simulink model "MATE_IEEE123Node"  (R2024b)
settings: Solver=FixedStepDiscrete  StartTime=0.0  StopTime=1  FixedStep=Ts  RelTol=1e-3
PostLoadFcn:
  | Ts=50e-6;init_IEEE123Node;
InitFcn:
  | Ts=50e-6;init_IEEE123Node;
values from neighbouring files (symbols this model uses):
  ft2km = 0.0003048    [init_IEEE123Node.m]
  loadcoeff = 1    [init_IEEE123Node.m]
  VsubL = 4.16 * 1000    (= 4160)    [init_IEEE123Node.m]
undefined symbols (not defined in the file or in its folder): MATE, MATERT, Pa1, Pa13, Pa14, Pa17, Pa18, Pa22, Pa24, Pa25, Pa29, Pa31, Pa32, Pa33, Pa34, Pa35, Pa37, Pa38, Pa39, Pa44, Pa46, Pa48, Pa50, Pa51, Pa52, Pa53, Pa57, Pa59, Pa6, Pa61, Pa67, Pa7, Pa70, Pa73, Pa8, Pa81, Pa82, Pa83, Pa84, Pa85, Pa9, Pb10, Pb15, Pb2, Pb30, Pb33, Pb34, Pb35, Pb41, Pb42, Pb43, Pb47, Pb48, Pb57, Pb58, Pb60, Pb65, Pb66, Pb68, Pb71 ... (+121)
libraries: simetranss x259, ee_lib x93, fl_lib x67, nesl_utility x67, simetran x2
(part 1 of 4)
settings Model: ARTEMISmethode_block_infos=$$__separator__$$  Creator=Kyle
settings SolverCC: AlgebraicLoopSolver=TrustRegion
settings DataIOCC: LimitDataPoints=on  SaveFormat=Array  SaveOutput=off  SignalLogging=off  DSMLogging=off  SaveTime=off  ReturnWorkspaceOutputs=off
settings OptimizationCC: OptimizeBlockIOStorage=off  BufferReuse=off  GlobalBufferReuse=off  ExpressionFolding=off  LocalBlockOutputs=off  LifeSpan=inf
settings DebuggingCC: ReadBeforeWriteMsg=DisableAll  WriteAfterWriteMsg=DisableAll  WriteAfterReadMsg=DisableAll  SolverPrmCheckMsg=warning  UnconnectedInputMsg=warning  UnconnectedOutputMsg=warning  UnconnectedLineMsg=warning  AllowSymbolicDim=off  SFUnexpectedBacktrackingDiag=warning  SFNoUnconditionalDefaultTransitionDiag=warning  SFExecutionAtInitializationDiag=none  ArithmeticOperatorsInVariantConditions=warning
settings HardwareCC: ProdBitPerPointer=32  ProdBitPerSizeT=32  ProdBitPerPtrDiffT=32  ProdLargestAtomicFloat=None  ProdIntDivRoundTo=Undefined  ProdEndianess=Unspecified  ProdWordSize=32  ProdHWDeviceType=32-bit Generic
settings ModelReferenceCC: EnableRefExpFcnMdlSchedulingChecks=on  PropagateSignalLabelsOutOfModel=off
settings SFSimCC: SimUseLocalCustomCode=off  CustomCodeUndefinedFunction=UseInterfaceOnly
settings RTWCC: RTWUseLocalCustomCode=off  GPUComputeCapability=3.5
settings CodeAppCC: StateflowObjectComments=on
settings GRTTargetCC: TargetLangStandard=C89/C90 (ANSI)  CombineOutputUpdateFcns=off  GRTInterface=on
settings ConfigComp: CovMetricSettings=dw  CovSaveCumulativeToWorkspaceVar=on  CovSaveSingleToWorkspaceVar=on  CovExternalEMLEnable=off
settings SimscapeCC: SimscapeNormalizeSystem=off

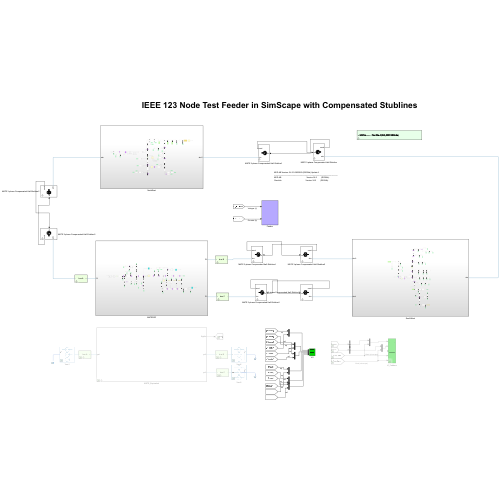
[thumbnail: Simulink's stored preview of the top-level diagram]
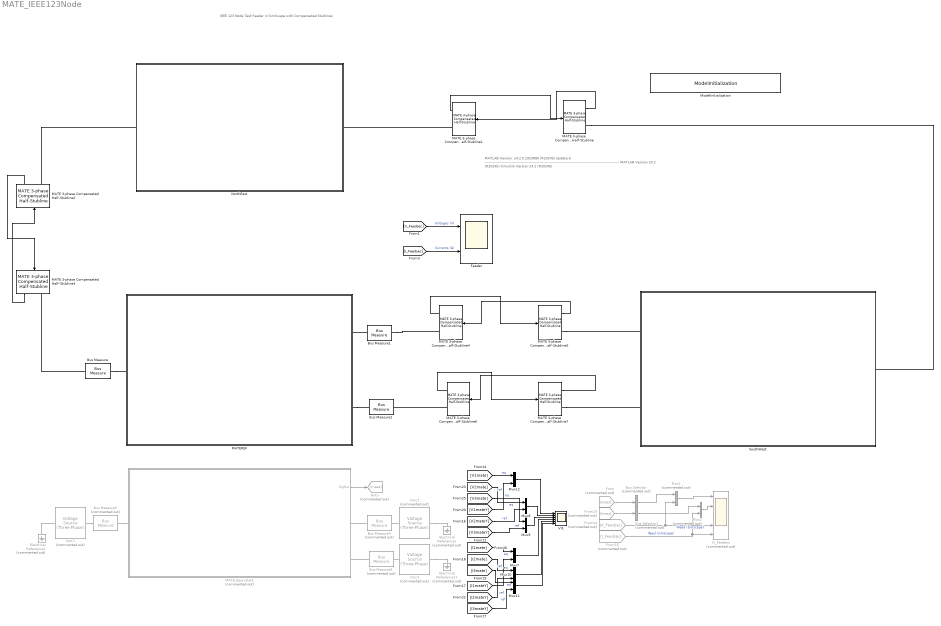
== system MATE_IEEE123Node ==
  note: MATLAB Version: 24.2.0.2923080 (R2024b) Update 6  -----------------------------------------------------------------------------------------------------
      | MATLAB                                                Version 24.2        (R2024b)
      |  Simulink                                              Version 24.2        (R2024b)
  note: IEEE 123 Node Test Feeder in SimScape with Compensated Stublines
  Bus Selector : BusSelector  Commented=on  OutputSignals=Voltage:_5_CV_xfo,Voltage:_6_CV_xfo,Voltage:_7_CV_xfo  OutputAsBus=on
  Bus Selector1 : BusSelector  Commented=on  OutputSignals=current:_11_CV_xfo,current:_12_CV_xfo,current:_13_CV_xfo  OutputAsBus=on
  Bus Measure : simetranss/Measure/Bus Measure  VoltageMeasurement=phase-to-ground  SetLabelV=on  LabelV=V1mateY  Vpu=off  VpuLL=off  CurrentMeasurement=yes  SetLabelI=on  LabelI=I1mateY  Ipu=off  Pbase=100e6  Vbase=500e3  bnumber=A  dis=off
  Bus Measure1 : simetranss/Measure/Bus Measure  VoltageMeasurement=phase-to-ground  SetLabelV=on  LabelV=V2mateY  Vpu=off  VpuLL=off  CurrentMeasurement=yes  SetLabelI=on  LabelI=I2mateY  Ipu=off  Pbase=100e6  Vbase=500e3  bnumber=B  dis=off
  Bus Measure2 : simetranss/Measure/Bus Measure  VoltageMeasurement=phase-to-ground  SetLabelV=on  LabelV=V3mateY  Vpu=off  VpuLL=off  CurrentMeasurement=yes  SetLabelI=on  LabelI=I3mateY  Ipu=off  Pbase=100e6  Vbase=500e3  bnumber=C  dis=off
  Bus Measure3 : simetranss/Measure/Bus Measure  Commented=on  VoltageMeasurement=phase-to-ground  SetLabelV=on  LabelV=V1mate  Vpu=off  VpuLL=off  CurrentMeasurement=yes  SetLabelI=on  LabelI=I1mate  Ipu=off  Pbase=100e6  Vbase=500e3  bnumber=A  dis=off
  Bus Measure4 : simetranss/Measure/Bus Measure  Commented=on  VoltageMeasurement=phase-to-ground  SetLabelV=on  LabelV=V2mate  Vpu=off  VpuLL=off  CurrentMeasurement=yes  SetLabelI=on  LabelI=I2mate  Ipu=off  Pbase=100e6  Vbase=500e3  bnumber=B  dis=off
  Bus Measure5 : simetranss/Measure/Bus Measure  Commented=on  VoltageMeasurement=phase-to-ground  SetLabelV=on  LabelV=V3mate  Vpu=off  VpuLL=off  CurrentMeasurement=yes  SetLabelI=on  LabelI=I3mate  Ipu=off  Pbase=100e6  Vbase=500e3  bnumber=C  dis=off
  Electrical Reference1 : fl_lib/Electrical/Electrical Elements/Electrical Reference  Commented=on
  Electrical Reference11 : fl_lib/Electrical/Electrical Elements/Electrical Reference  Commented=on
  Electrical Reference2 : fl_lib/Electrical/Electrical Elements/Electrical Reference  Commented=on
  Feeder : Scope  NumInputPorts=2
  From : From  Commented=on  GotoTag=meas
  From13 : From  Commented=on  GotoTag=meas
  From14 : From  Commented=on  GotoTag=V_Feedsec  TagVisibility=global
  From15 : From  Commented=on  GotoTag=I_Feedsec  TagVisibility=global
  Goto : Goto  Commented=on  GotoTag=meas
  MATE 3-phase Compensated Half-Stubline : simetranss/Network decoupling/MATE 3-phase Compensated Half-Stubline  stype=3-phase coupled line (1 mode)  FF=60  RR=[ 0.4615 0.1535 0.1580; 0.1535 0.4576 0.1560; 0.1580 0.1560 0.4666]*0.621371  LL=[1.0651 0.3849 0.4236; 0.3849 1.0780 0.5017; 0.4236 0.5017 1.0482]/(2*pi*60)*0.621371  CC=[ 5.3971 -0.6982 -1.1645; -0.6982 5.6765 -1.8319; -1.1645 -1.8319 5.9809]*1e-6/(2*pi*60)*0.621371  len=1000*ft2km  Ts=Ts  comp=on  stdel=off
  MATE 3-phase Compensated Half-Stubline1 : simetranss/Network decoupling/MATE 3-phase Compensated Half-Stubline  stype=3-phase coupled line (1 mode)  FF=60  RR=[ 0.4615 0.1535 0.1580; 0.1535 0.4576 0.1560; 0.1580 0.1560 0.4666]*0.621371  LL=[1.0651 0.3849 0.4236; 0.3849 1.0780 0.5017; 0.4236 0.5017 1.0482]/(2*pi*60)*0.621371  CC=[ 5.3971 -0.6982 -1.1645; -0.6982 5.6765 -1.8319; -1.1645 -1.8319 5.9809]*1e-6/(2*pi*60)*0.621371  len=1000*ft2km  Ts=Ts  comp=off  stdel=off
  MATE 3-phase Compensated Half-Stubline2 : simetranss/Network decoupling/MATE 3-phase Compensated Half-Stubline  stype=3-phase coupled line (1 mode)  FF=60  RR=[ 0.4666 0.1580 0.1560; 0.1580 0.4615 0.1535; 0.1560 0.1535 0.4576]*0.621371  LL=[ 1.0482 0.4236 0.5017; 0.4236 1.0651 0.3849; 0.5017 0.3849 1.0780]/(2*pi*60)*0.621371  CC=[ 5.9809 -1.1645 -1.8319; -1.1645 5.3971 -0.6982; -1.8319 -0.6982 5.6765]*1e-6/(2*pi*60)*0.621371  len=825*ft2km  Ts=Ts  comp=on  stdel=off
  MATE 3-phase Compensated Half-Stubline3 : simetranss/Network decoupling/MATE 3-phase Compensated Half-Stubline  stype=3-phase coupled line (1 mode)  FF=60  RR=[ 0.4666 0.1580 0.1560; 0.1580 0.4615 0.1535; 0.1560 0.1535 0.4576]*0.621371  LL=[ 1.0482 0.4236 0.5017; 0.4236 1.0651 0.3849; 0.5017 0.3849 1.0780]/(2*pi*60)*0.621371  CC=[ 5.9809 -1.1645 -1.8319; -1.1645 5.3971 -0.6982; -1.8319 -0.6982 5.6765]*1e-6/(2*pi*60)*0.621371  len=825*ft2km  Ts=Ts  comp=off  stdel=off
  MATE 3-phase Compensated Half-Stubline4 : simetranss/Network decoupling/MATE 3-phase Compensated Half-Stubline  stype=3-phase coupled line (1 mode)  FF=60  RR=[ 0.4615 0.1535 0.1580; 0.1535 0.4576 0.1560; 0.1580 0.1560 0.4666]*0.621371  LL=[1.0651 0.3849 0.4236; 0.3849 1.0780 0.5017; 0.4236 0.5017 1.0482]/(2*pi*60)*0.621371  CC=[ 5.3971 -0.6982 -1.1645; -0.6982 5.6765 -1.8319; -1.1645 -1.8319 5.9809]*1e-6/(2*pi*60)*0.621371  len=750*ft2km  Ts=Ts  comp=off  stdel=off
  MATE 3-phase Compensated Half-Stubline5 : simetranss/Network decoupling/MATE 3-phase Compensated Half-Stubline  stype=3-phase coupled line (1 mode)  FF=60  RR=[ 0.4615 0.1535 0.1580; 0.1535 0.4576 0.1560; 0.1580 0.1560 0.4666]*0.621371  LL=[1.0651 0.3849 0.4236; 0.3849 1.0780 0.5017; 0.4236 0.5017 1.0482]/(2*pi*60)*0.621371  CC=[ 5.3971 -0.6982 -1.1645; -0.6982 5.6765 -1.8319; -1.1645 -1.8319 5.9809]*1e-6/(2*pi*60)*0.621371  len=750*ft2km  Ts=Ts  comp=on  stdel=off
  MATE 3-phase Compensated Half-Stubline6 : simetranss/Network decoupling/MATE 3-phase Compensated Half-Stubline  stype=3-phase coupled line (1 mode)  FF=60  RR=[ 0.4615 0.1535 0.1580; 0.1535 0.4576 0.1560; 0.1580 0.1560 0.4666]*0.621371  LL=[1.0651 0.3849 0.4236; 0.3849 1.0780 0.5017; 0.4236 0.5017 1.0482]/(2*pi*60)*0.621371  CC=[ 5.3971 -0.6982 -1.1645; -0.6982 5.6765 -1.8319; -1.1645 -1.8319 5.9809]*1e-6/(2*pi*60)*0.621371  len=700*ft2km  Ts=Ts  comp=on  stdel=off
  MATE 3-phase Compensated Half-Stubline7 : simetranss/Network decoupling/MATE 3-phase Compensated Half-Stubline  stype=3-phase coupled line (1 mode)  FF=60  RR=[ 0.4615 0.1535 0.1580; 0.1535 0.4576 0.1560; 0.1580 0.1560 0.4666]*0.621371  LL=[1.0651 0.3849 0.4236; 0.3849 1.0780 0.5017; 0.4236 0.5017 1.0482]/(2*pi*60)*0.621371  CC=[ 5.3971 -0.6982 -1.1645; -0.6982 5.6765 -1.8319; -1.1645 -1.8319 5.9809]*1e-6/(2*pi*60)*0.621371  len=700*ft2km  Ts=Ts  comp=off  stdel=off
  MATEREF : Subsystem
  MATE_Equivalent : Subsystem  Commented=on  mask(MATE object){MATE=MATE, MATERT=MATERT}
      mask prompts: MATE "General MATE data structure name"; MATERT "MATE S-function parameter"
      mask help:
      | MATE Object (Multu-Area Thevenin Equivalent) is a generalized EMT-type branch.
      | They can be used to build equivalent circuit with less solver apparent nodes.
      mask DialogControl Control2 Prompt: Generate MATE equations
      mask DialogControl Control2 Callback:
      | [MATE, MATERT]= MakeMate('Simscape_IEEE123_oneThird/MATEREF', 1);
      | assignin("base","MATE",MATE);
      | assignin("base","MATERT",MATERT);
  ModelInitialization : simetranss/Usefulls/ModelInitialization  InitFcnX=Ts=50e-6;init_IEEE123Node;  prel=off  posl=on  inif=on  strf=off
  Mux1 : Mux  Commented=on  Inputs=2
  Mux{7..12} (6 alike) : Mux  Inputs=2
  Mux2 : Mux  Commented=on  Inputs=2
  NorthEast : Subsystem
  SouthWest : Subsystem
  VI1 : Scope  NumInputPorts=6
  VI_Fedders : Scope  Commented=on  NumInputPorts=5
  Vsrc1 : ee_lib/Sources/Voltage Source (Three-Phase)  Commented=on  vline_rms=4160 V  shift=0 deg  freq=60 Hz  impedance_option=4  SShortCircuit=1e6 A*V  XR=15  R=0.1 Ohm  L=1e-3 H  harmonic_option=0  harmonic_orders=[5, 7, 11, 13]  harmonic_ratios=[.1, .1, .1, .1]  G_parasitic=0 1/Ohm  I_specify=off  I_priority=None  I=[0, 0, 0] A  I_nominal_specify=off  I_nominal_value=1  I_nominal_unit=A
  Vsrc2 : ee_lib/Sources/Voltage Source (Three-Phase)  Commented=on  vline_rms=4160 V  shift=15 deg  freq=60 Hz  impedance_option=4  SShortCircuit=1e6 A*V  XR=15  R=0.1 Ohm  L=1e-3 H  harmonic_option=0  harmonic_orders=[5, 7, 11, 13]  harmonic_ratios=[.1, .1, .1, .1]  G_parasitic=0 1/Ohm  I_specify=off  I_priority=None  I=[0, 0, 0] A  I_nominal_specify=off  I_nominal_value=1  I_nominal_unit=A
  Vsrc3 : ee_lib/Sources/Voltage Source (Three-Phase)  Commented=on  vline_rms=4160 V  shift=30 deg  freq=60 Hz  impedance_option=4  SShortCircuit=1e6 A*V  XR=15  R=0.1 Ohm  L=1e-3 H  harmonic_option=0  harmonic_orders=[5, 7, 11, 13]  harmonic_ratios=[.1, .1, .1, .1]  G_parasitic=0 1/Ohm  I_specify=off  I_priority=None  I=[0, 0, 0] A  I_nominal_specify=off  I_nominal_value=1  I_nominal_unit=A
  wires:
  [I2mateY] -> Mux10/2  "ref"
  [I1mate] -> Mux7/1  "eq"
  From13/1 -> Bus Selector1/1
  From/1 -> Bus Selector/1
  Mux9/1 -> VI1/3
  [V2mate] -> Mux8/1  "eq"
  [V3mateY] -> Mux9/2  "ref"
  Bus Selector1/1 -> Mux2/1
  Mux11/1 -> VI1/6
  Mux12/1 -> VI1/1
  Mux10/1 -> VI1/5
  [I2mate] -> Mux10/1  "eq"
  [V3mate] -> Mux9/1  "eq"
  Mux7/1 -> VI1/4
  [V1mate] -> Mux12/1  "eq"
  [I3mateY] -> Mux11/2  "ref"
  [I3mate] -> Mux11/1  "eq"
  [I1mateY] -> Mux7/2  "ref"
  From14/1 -> Mux1/2, VI_Fedders/4  "Vfeed (simscape)"
  Mux1/1 -> VI_Fedders/1
  Mux8/1 -> VI1/2
  Bus Selector/1 -> Mux1/1
  Mux2/1 -> VI_Fedders/2
  [V1mateY] -> Mux12/2  "ref"
  From15/1 -> Mux2/2, VI_Fedders/5  "Ifeed (simscape)"
  MATE_Equivalent/1(SigOut) -> Goto/1
  [V2mateY] -> Mux8/2  "ref"
  MATE 3-phase Compensated Half-Stubline/1 -> MATE 3-phase Compensated Half-Stubline1/1
  MATE 3-phase Compensated Half-Stubline1/1 -> MATE 3-phase Compensated Half-Stubline/1
  MATE 3-phase Compensated Half-Stubline2/1 -> MATE 3-phase Compensated Half-Stubline3/1
  MATE 3-phase Compensated Half-Stubline3/1 -> MATE 3-phase Compensated Half-Stubline2/1
  MATE 3-phase Compensated Half-Stubline4/1 -> MATE 3-phase Compensated Half-Stubline5/1
  MATE 3-phase Compensated Half-Stubline5/1 -> MATE 3-phase Compensated Half-Stubline4/1
  MATE 3-phase Compensated Half-Stubline6/1 -> MATE 3-phase Compensated Half-Stubline7/1
  MATE 3-phase Compensated Half-Stubline7/1 -> MATE 3-phase Compensated Half-Stubline6/1
  [V_Feedsec] -> Feeder/1  "Voltages (V)"
  [I_Feedsec] -> Feeder/2  "Currents (A)"
  connections:
  MATE 3-phase Compensated Half-Stubline6/RConn1 -- Bus Measure2/RConn1
  Bus Measure1/RConn1 -- MATE 3-phase Compensated Half-Stubline4/RConn1
  Bus Measure/RConn1 -- MATE 3-phase Compensated Half-Stubline3/RConn1
  Bus Measure/LConn1 -- MATEREF/LConn1
  MATEREF/RConn2 -- Bus Measure2/LConn1
  Vsrc3/LConn1 -- Electrical Reference11/LConn1
  Vsrc1/LConn1 -- Electrical Reference2/LConn1
  Vsrc3/RConn1 -- Bus Measure5/RConn1
  Vsrc2/LConn1 -- Electrical Reference1/LConn1
  Bus Measure1/LConn1 -- MATEREF/RConn1
  MATE 3-phase Compensated Half-Stubline1/RConn1 -- NorthEast/RConn1
  MATE 3-phase Compensated Half-Stubline/RConn1 -- SouthWest/RConn1
  MATE 3-phase Compensated Half-Stubline5/RConn1 -- SouthWest/LConn1
  MATE 3-phase Compensated Half-Stubline7/RConn1 -- SouthWest/LConn2
  Bus Measure3/LConn1 -- MATE_Equivalent/LConn1
  Bus Measure4/LConn1 -- MATE_Equivalent/RConn1
  NorthEast/LConn1 -- MATE 3-phase Compensated Half-Stubline2/RConn1
  Vsrc1/RConn1 -- Bus Measure3/RConn1
  Vsrc2/RConn1 -- Bus Measure4/RConn1
  Bus Measure5/LConn1 -- MATE_Equivalent/RConn2

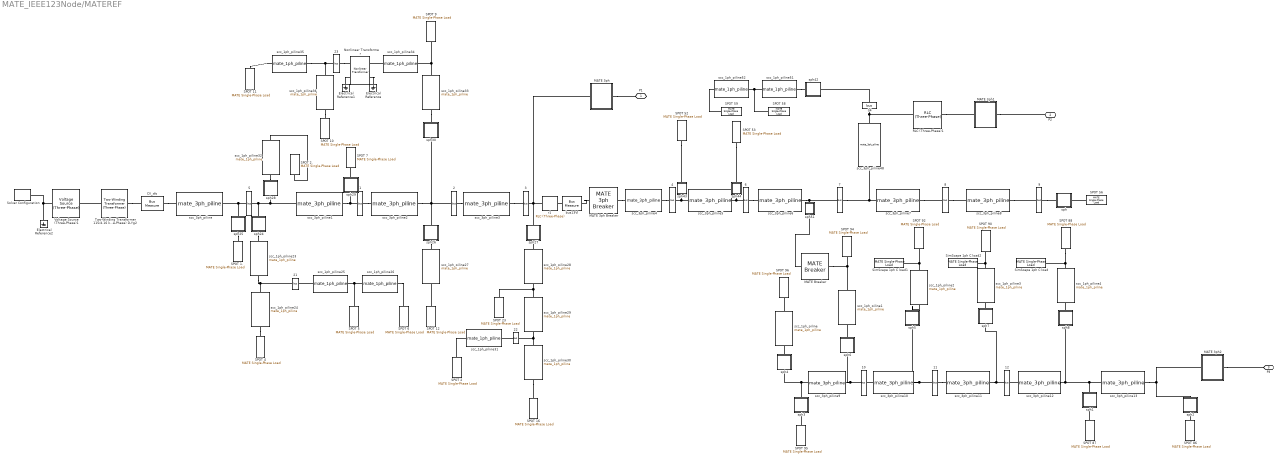
== system MATE_IEEE123Node/MATEREF ==
  1 : simetranss/Measure/bus  bn=7
      settings: AttributesFormatString=Bus %<bn>
  10 : simetranss/Measure/bus  bn=93
      settings: AttributesFormatString=Bus %<bn>
  11 : simetranss/Measure/bus  bn=91
      settings: AttributesFormatString=Bus %<bn>
  12 : simetranss/Measure/bus  bn=89
      settings: AttributesFormatString=Bus %<bn>
  2 : simetranss/Measure/bus  bn=8
      settings: AttributesFormatString=Bus %<bn>
  21 : simetranss/Measure/bus  bn=3
      settings: AttributesFormatString=Bus %<bn>
  22 : simetranss/Measure/bus  bn=15
      settings: AttributesFormatString=Bus %<bn>
  23 : simetranss/Measure/bus  bn=14
      settings: AttributesFormatString=Bus %<bn>
  3 : simetranss/Measure/bus  bn=13
      settings: AttributesFormatString=Bus %<bn>
  34 : simetranss/Measure/bus  bn=57
      settings: AttributesFormatString=Bus %<bn>
  4 : simetranss/Measure/bus  bn=52
      settings: AttributesFormatString=Bus %<bn>
  5 : simetranss/Measure/bus  bn=1
      settings: AttributesFormatString=Bus %<bn>
  6 : simetranss/Measure/bus  bn=53
      settings: AttributesFormatString=Bus %<bn>
  7 : simetranss/Measure/bus  bn=54
      settings: AttributesFormatString=Bus %<bn>
  8 : simetranss/Measure/bus  bn=55
      settings: AttributesFormatString=Bus %<bn>
  9 : simetranss/Measure/bus  bn=56
      settings: AttributesFormatString=Bus %<bn>
  CV_xfo : simetranss/Measure/Bus Measure  VoltageMeasurement=phase-to-ground  SetLabelV=on  LabelV=V_Feedsec  Vpu=off  VpuLL=off  CurrentMeasurement=yes  SetLabelI=on  LabelI=I_Feedsec  Ipu=off  Pbase=100e6  Vbase=500e3  bnumber=0  dis=off
  Electrical Reference : fl_lib/Electrical/Electrical Elements/Electrical Reference
  Electrical Reference1 : fl_lib/Electrical/Electrical Elements/Electrical Reference
  Electrical Reference2 : fl_lib/Electrical/Electrical Elements/Electrical Reference
  MATE 3ph : Subsystem  mask(MATE Node (3-phase)){bn=1, it=auto, Rse=1e-4, Rsh=1e9}
      mask prompts: bn "MATE node number"; it "Interface type"; Rse "Series resistance (Ohms)"; Rsh "Shunt resistance (Ohms)"
      mask help:
      | MATE interface for Single-Line Diagram SimScape model.
      |
      | This block is used to interface a MATE reduced set of block to a main circuit.
      | 'MATE' port must be connected toward the MATE reduced network.
      | 'Main' port must be connected toward the main (unreduced) network)
      settings: AttributesFormatString=# %<bn>
      mask TypeOptions it: auto | Thevenin | Norton
      mask Display: disp(['3ph' 10 10 10])
  MATE 3ph Breaker : simetranss/Switches/MATE 3ph Breaker  InitialState=closed  SwitchA=off  SwitchB=off  SwitchC=off  SwitchTimes="[1/60  5/60]"  External=off  BreakerResistance=0.01  Roff=0  SnubberResistance=1e6  SnubberCapacitance=inf
  MATE 3ph1 : Subsystem  mask(MATE Node (3-phase)){bn=2, it=auto, Rse=1e-4, Rsh=1e9}
      mask prompts: bn "MATE node number"; it "Interface type"; Rse "Series resistance (Ohms)"; Rsh "Shunt resistance (Ohms)"
      mask help:
      | MATE interface for Single-Line Diagram SimScape model.
      |
      | This block is used to interface a MATE reduced set of block to a main circuit.
      | 'MATE' port must be connected toward the MATE reduced network.
      | 'Main' port must be connected toward the main (unreduced) network)
      settings: AttributesFormatString=# %<bn>
      mask TypeOptions it: auto | Thevenin | Norton
      mask Display: disp(['3ph' 10 10 10])
  MATE 3ph2 : Subsystem  mask(MATE Node (3-phase)){bn=3, it=auto, Rse=1e-4, Rsh=1e9}
      mask prompts: bn "MATE node number"; it "Interface type"; Rse "Series resistance (Ohms)"; Rsh "Shunt resistance (Ohms)"
      mask help:
      | MATE interface for Single-Line Diagram SimScape model.
      |
      | This block is used to interface a MATE reduced set of block to a main circuit.
      | 'MATE' port must be connected toward the MATE reduced network.
      | 'Main' port must be connected toward the main (unreduced) network)
      settings: AttributesFormatString=# %<bn>
      mask TypeOptions it: auto | Thevenin | Norton
      mask Display: disp(['3ph' 10 10 10])
  MATE Breaker : simetranss/Switches/MATE Breaker  InitialState=open  SwitchA=on  SwitchB=on  SwitchC=off  SwitchTimes="[1/60  5/60]"  External=off  BreakerResistance=0.01  Roff=1e6  SnubberResistance=1e6  SnubberCapacitance=inf
  Nonlinear Transformer : ee_lib/Passive/Transformers/Nonlinear Transformer  Nw=1  Nw2=1  winding_param_option=2  Req=0.01 Ohm  Leq=0.0001 H  R_1=0.001 Ohm  L_1=0.001 H  R_2=0.001 Ohm  L_2=0.001 H  averaging_period=0 s  R_m=50000 Ohm  parameterization_option=1  H_data=[0, 200, 400, 600, 800, 1000] A/m  B_data=[0, .81, 1.25, 1.42, 1.48, 1.49] T  length_effective=0.2 m  area_effective=2e-4 m^2  L=4e-2 H  L_sat=1e-2 H  current_data=[0, .4, .8, 1.2, 1.6, 2] A  magnetic_flux_data=[0, .161, .25, .284, .295, .299] .* 1e-3 Wb  magnetic_flux_sat=1.6e-04 Wb  dBdH0=0.005 T*m/A  B1=1.49 T  H1=1000 A/m  c=0.1  K=200 A/m  alpha=1e-4  interpolation_option=1  Leq_i0=0 A  L1_i0=0 A  L2_i0=0 A  x0_option=1  i_L0=0 A  phi0=0 Wb  B0=0 T  H0=0 A/m  Leq_g=1e-9 1/Ohm  L1_g=1e-9 1/Ohm  L2_g=1e-9 1/Ohm
      settings: InternalSimscapePortConfiguration="{\"Bottom\":[],\"Left\":[{\"id\":\"p1\",\"label\":\"1+\",\"type\":\"foundation.electrical.electrical\"},{\"id\":\"n1\",\"label\":\"1-\",\"type\":\"foundation.electrical.electrical\"}],\"Right\":[{\"id\":\"p2\",\"label\":\"2+\",\"type\":\"foundation.electrical.electrical\"},{\"id\":\"n2\",\"label\":\"2-\",\"type\":\"foundation.electrical.electrical\"}],\"Top\":[]}"
  RLC (Three-Phase)1 : ee_lib/Passive/RLC Assemblies/RLC (Three-Phase)  port_option=ee.enum.threePhasePort.composite  component_structure=ee.enum.rlc.structure.SeriesRL  R=1e-2 Ohm  L=1e-6 H  C=1e-6 F  R_parasitic=0 Ohm  G_parasitic=0 1/Ohm  IL_specify=off  IL_priority=High  IL=[0, 0, 0] A  IL_nominal_specify=off  IL_nominal_value=1  IL_nominal_unit=A  VC_specify=off  VC_priority=High  VC=[0, 0, 0] V  VC_nominal_specify=off  VC_nominal_value=1  VC_nominal_unit=V
      settings: InternalSimscapePortConfiguration="{\"Bottom\":[],\"Left\":[{\"id\":\"N1\",\"label\":\"~1\",\"type\":\"foundation.electrical.three_phase\"}],\"Right\":[{\"id\":\"N2\",\"label\":\"~2\",\"type\":\"foundation.electrical.three_phase\"}],\"Top\":[]}"
  SPOT 1. : simetranss/Passive/MATE Single-Phase Load  Vabc=VsubL/sqrt(3)  Fn=60  typ=Series RL  Pabc=Pa1*loadcoeff  QLabc=Qa1*loadcoeff  QCabc="[190  ]*1e3"
  SPOT 10 : simetranss/Passive/MATE Single-Phase Load  Vabc=VsubL/sqrt(3)  Fn=60  typ=Series RL  Pabc=Pa8*loadcoeff  QLabc=Qa8*loadcoeff  QCabc="[190  ]*1e3"
  SPOT 11 : simetranss/Passive/MATE Single-Phase Load  Vabc=VsubL/sqrt(3)  Fn=60  typ=Series RL  Pabc=Pa9*loadcoeff  QLabc=Qa9*loadcoeff  QCabc="[190  ]*1e3"
  SPOT 12 : simetranss/Passive/MATE Single-Phase Load  Vabc=VsubL/sqrt(3)  Fn=60  typ=Series RL  Pabc=Pb10*loadcoeff  QLabc=Qb10*loadcoeff  QCabc="[190  ]*1e3"
  SPOT 16 : simetranss/Passive/MATE Single-Phase Load  Vabc=VsubL/sqrt(3)  Fn=60  typ=Series RL  Pabc=Pc11*loadcoeff  QLabc=Qc11*loadcoeff  QCabc="[190  ]*1e3"
  SPOT 2 : simetranss/Passive/MATE Single-Phase Load  Vabc=VsubL/sqrt(3)  Fn=60  typ=Series RL  Pabc=Pc12*loadcoeff  QLabc=Qc12*loadcoeff  QCabc="[190  ]*1e3"
  SPOT 2. : simetranss/Passive/MATE Single-Phase Load  Vabc=VsubL/sqrt(3)  Fn=60  typ=Series RL  Pabc=Pb2*loadcoeff  QLabc=Qb2*loadcoeff  QCabc="[190  ]*1e3"
  SPOT 23 : simetranss/Passive/MATE Single-Phase Load  Vabc=VsubL/sqrt(3)  Fn=60  typ=Series RL  Pabc=Pc11*loadcoeff  QLabc=Qc11*loadcoeff  QCabc="[190  ]*1e3"
  SPOT 4 : simetranss/Passive/MATE Single-Phase Load  Vabc=VsubL/sqrt(3)  Fn=60  typ=Series RL  Pabc=Pc3*loadcoeff  QLabc=Qc3*loadcoeff  QCabc="[190  ]*1e3"
  SPOT 5 : simetranss/Passive/MATE Single-Phase Load  Vabc=VsubL/sqrt(3)  Fn=60  typ=Series RL  Pabc=Pc4*loadcoeff  QLabc=Qc4*loadcoeff  QCabc="[190  ]*1e3"
  SPOT 52 : simetranss/Passive/MATE Single-Phase Load  Vabc=VsubL/sqrt(3)  Fn=60  typ=Series RL  Pabc=Pa38*loadcoeff  QLabc=Qa38*loadcoeff  QCabc="[190  ]*1e3"
  SPOT 53 : simetranss/Passive/MATE Single-Phase Load  Vabc=VsubL/sqrt(3)  Fn=60  typ=Series RL  Pabc=Pa39*loadcoeff  QLabc=Qa39*loadcoeff  QCabc="[190  ]*1e3"
  SPOT 56 : simetranss/Passive/MATE Single-Phase Load  Vabc=VsubL/sqrt(3)  Fn=60  typ=Series RL  Pabc=Pb41*loadcoeff  QLabc=Qb41*loadcoeff  QCabc="[190  ]*1e3"
  SPOT 58 : simetranss/Passive/MATE Single-Phase Load  Vabc=VsubL/sqrt(3)  Fn=60  typ=Series RL  Pabc=Pb42*loadcoeff  QLabc=Qb42*loadcoeff  QCabc="[190  ]*1e3"
  SPOT 59 : simetranss/Passive/MATE Single-Phase Load  Vabc=VsubL/sqrt(3)  Fn=60  typ=Series RL  Pabc=Pb43*loadcoeff  QLabc=Qb43*loadcoeff  QCabc="[190  ]*1e3"
  SPOT 6 : simetranss/Passive/MATE Single-Phase Load  Vabc=VsubL/sqrt(3)  Fn=60  typ=Series RL  Pabc=Pc5*loadcoeff  QLabc=Qc5*loadcoeff  QCabc="[190  ]*1e3"
  SPOT 7 : simetranss/Passive/MATE Single-Phase Load  Vabc=VsubL/sqrt(3)  Fn=60  typ=Series RL  Pabc=Pa6*loadcoeff  QLabc=Qa6*loadcoeff  QCabc="[190  ]*1e3"
  SPOT 86 : simetranss/Passive/MATE Single-Phase Load  Vabc=VsubL/sqrt(3)  Fn=60  typ=Series RL  Pabc=Pb65*loadcoeff  QLabc=Qb65*loadcoeff  QCabc="[190  ]*1e3"
  SPOT 87 : simetranss/Passive/MATE Single-Phase Load  Vabc=VsubL/sqrt(3)  Fn=60  typ=Series RL  Pabc=Pb66*loadcoeff  QLabc=Qb66*loadcoeff  QCabc="[190  ]*1e3"
  SPOT 88 : simetranss/Passive/MATE Single-Phase Load  Vabc=VsubL/sqrt(3)  Fn=60  typ=Series RL  Pabc=Pa67*loadcoeff  QLabc=Qa67*loadcoeff  QCabc="[190  ]*1e3"
  SPOT 9 : simetranss/Passive/MATE Single-Phase Load  Vabc=VsubL/sqrt(3)  Fn=60  typ=Series RL  Pabc=Pa7*loadcoeff  QLabc=Qa7*loadcoeff  QCabc="[190  ]*1e3"
  SPOT 90 : simetranss/Passive/MATE Single-Phase Load  Vabc=VsubL/sqrt(3)  Fn=60  typ=Series RL  Pabc=Pb68*loadcoeff  QLabc=Qb68*loadcoeff  QCabc="[190  ]*1e3"
  SPOT 92 : simetranss/Passive/MATE Single-Phase Load  Vabc=VsubL/sqrt(3)  Fn=60  typ=Series RL  Pabc=Pc69*loadcoeff  QLabc=Qc69*loadcoeff  QCabc="[190  ]*1e3"
  SPOT 94 : simetranss/Passive/MATE Single-Phase Load  Vabc=VsubL/sqrt(3)  Fn=60  typ=Series RL  Pabc=Pa70*loadcoeff  QLabc=Qa70*loadcoeff  QCabc="[190  ]*1e3"
  SPOT 95 : simetranss/Passive/MATE Single-Phase Load  Vabc=VsubL/sqrt(3)  Fn=60  typ=Series RL  Pabc=Pb71*loadcoeff  QLabc=Qb71*loadcoeff  QCabc="[190  ]*1e3"
  SPOT 96 : simetranss/Passive/MATE Single-Phase Load  Vabc=VsubL/sqrt(3)  Fn=60  typ=Series RL  Pabc=Pb72*loadcoeff  QLabc=Qb72*loadcoeff  QCabc="[190  ]*1e3"
  SimScape 1ph C load : simetranss/Passive/MATE Single-Phase Load  Vabc=4160/sqrt(3)  Fn=60  typ=Capacitance  Pabc=[160 ]*1e3  QLabc=[ 90]*1e3  QCabc=100e3
  SimScape 1ph C load1 : simetranss/Passive/MATE Single-Phase Load  Vabc=VsubL/sqrt(3)  Fn=60  typ=Capacitance  Pabc=[160 ]*1e3  QLabc=[ 90]*1e3  QCabc=50e3
  SimScape 1ph C load2 : simetranss/Passive/MATE Single-Phase Load  Vabc=VsubL/sqrt(3)  Fn=60  typ=Capacitance  Pabc=[160 ]*1e3  QLabc=[ 90]*1e3  QCabc=50e3
  Solver Configuration : nesl_utility/Solver Configuration  PhysicalDomain=network_engine_domain  SubClassName=solver  LeftPortType=input  RightPortType=generic  Tones=[]  Harmonics=[]  SimulateNoise=off  Profile=off  UseLocalSampling=off  EnableSwitchedLinearOptims=on  FrequencyDomain=off  UseCCode=off  RelTol=0.001  AbsTol=0.001  MinStep=1e-09  ToWorkspace=off  RevertToSquareIcSolve=off  NumHomotopyIterations=100  PhasorMode=off  PhasorModeNumHarmonics=1  ConsistencySolver=NEWTON_XTOL_AFTER_FTOL  IndexReductionMethod=None  DoDC=off  ResidualTolerance=1e-09  ConsistencyTolSource=GLOBAL  ConsistencyAbsTol=0.001  ConsistencyRelTol=0.001  ConsistencyTolFactor=0.1  UseLocalSolver=on  LocalSolverChoice=NE_PARTITIONING_ADVANCER  ResolveIndetEquations=off  FunctionEvalNumThread=1  LocalSolverSampleTime=Ts  DoFixedCost=on  MaxNonlinIter=1  MaxModeIter=2  ComputeImpulses=off  ImpulseIterations=2  LinearAlgebra=auto  LinearAlgebraNumThread=0  EquationFormulation=NE_TIME_EF  DelaysMemoryBudget=1024  AutomaticFiltering=on  FilteringTimeConstant=0.001  PartitionStorageMethod=AS_NEEDED  PartitionMemoryBudget=1024  PartitionMethod=ROBUST  MultibodyUseLocalSolver=off  MultibodyLocalSolverChoice=ODE1  MultibodyLocalSolverSampleTime=0.001
  Two-Winding Transformer 115/4.16 kV (Three-Phase) D-Yg2 : ee_lib/Passive/Transformers/Two-Winding Transformer (Three-Phase)  SRated=6e6 A*V  FRated=60 Hz  Winding1Connection=ee.enum.windingconnection.delta1  VRated1=115e3 V  Winding2Connection=ee.enum.windingconnection.Yg  VRated2=4160 V  CoreType=ee.enum.coretype.fivelimb  pu_Rw1=0.01/2  pu_Rw2=0.01/2  leakage_reactance_option=ee.enum.transformer_leakage.include  pu_Xl1=0.08/2  pu_Xl2=0.08/2  magnetizing_resistance_option=ee.enum.transformer_magnetizingResistance.include  pu_Rm=100  magnetizing_reactance_option=ee.enum.transformer_magnetizingReactance.include  saturation_option=ee.enum.transformer_saturation.exclude  pu_Xm=100  current_data=[0, .002, 1, 2]  magnetic_flux_data=[0, 1.2, 1.5, 1.51]  pu_X0=5000  i1_specify=off  i1_priority=None  i1=[0, 0, 0] A  i1_nominal_specify=off  i1_nominal_value=1  i1_nominal_unit=A  i2_specify=off  i2_priority=None  i2=[0, 0, 0] A  i2_nominal_specify=off  i2_nominal_value=1  i2_nominal_unit=A  phi_specify=off  phi_priority=None  phi=[0, 0, 0]  phi_nominal_specify=off  phi_nominal_value=1  phi_nominal_unit=1  power_dissipated_specify=off  power_dissipated_priority=None  power_dissipated=0 W  power_dissipated_nominal_specify=off  power_dissipated_nominal_value=1  power_dissipated_nominal_unit=W
      settings: InternalSimscapePortConfiguration="{\"Bottom\":[],\"Left\":[{\"id\":\"N1\",\"label\":\"~1\",\"type\":\"foundation.electrical.three_phase\"}],\"Right\":[{\"id\":\"N2\",\"label\":\"~2\",\"type\":\"foundation.electrical.three_phase\"}],\"Top\":[]}"
  Voltage Source (Three-Phase)1 : ee_lib/Sources/Voltage Source (Three-Phase)  vline_rms=115e3 V  shift=90 deg  freq=60 Hz  impedance_option=2  SShortCircuit=1e6 A*V  XR=15  R=0.001 Ohm  L=3.97e-4 H  harmonic_option=0  harmonic_orders=[5, 7, 11, 13]  harmonic_ratios=[.1, .1, .1, .1]  G_parasitic=0 1/Ohm  I_specify=off  I_priority=None  I=[0, 0, 0] A  I_nominal_specify=off  I_nominal_value=1  I_nominal_unit=A
  bus13VI : simetranss/Measure/Bus Measure  VoltageMeasurement=phase-to-ground  SetLabelV=on  LabelV=V13  Vpu=off  VpuLL=off  CurrentMeasurement=yes  SetLabelI=on  LabelI=I13  Ipu=off  Pbase=100e6  Vbase=500e3  bnumber=13  dis=off
  r1 : ee_lib/Passive/RLC Assemblies/RLC (Three-Phase)  port_option=ee.enum.threePhasePort.composite  component_structure=ee.enum.rlc.structure.R  R=1e-3 Ohm  L=1e-3 H  C=1e-6 F  R_parasitic=0 Ohm  G_parasitic=0 1/Ohm  IL_specify=off  IL_priority=High  IL=[0, 0, 0] A  IL_nominal_specify=off  IL_nominal_value=1  IL_nominal_unit=A  VC_specify=off  VC_priority=High  VC=[0, 0, 0] V  VC_nominal_specify=off  VC_nominal_value=1  VC_nominal_unit=V
      settings: InternalSimscapePortConfiguration="{\"Bottom\":[],\"Left\":[{\"id\":\"N1\",\"label\":\"~1\",\"type\":\"foundation.electrical.three_phase\"}],\"Right\":[{\"id\":\"N2\",\"label\":\"~2\",\"type\":\"foundation.electrical.three_phase\"}],\"Top\":[]}"
  scc_1ph_piline : simetranss/Lines/mate_1ph_piline  FF=60  conf=config 10  lenfeet=200  dmi=off  RR1=0.8  LL1=0.002  CC1=7e-9  lenkm=300*ft2km
  scc_1ph_piline1 : simetranss/Lines/mate_1ph_piline  FF=60  conf=config 9  lenfeet=275  dmi=off  RR1=0.8  LL1=0.002  CC1=7e-9  lenkm=300*ft2km
  scc_1ph_piline2 : simetranss/Lines/mate_1ph_piline  FF=60  conf=config 11  lenfeet=300  dmi=off  RR1=0.8  LL1=0.002  CC1=7e-9  lenkm=300*ft2km
  scc_1ph_piline23 : simetranss/Lines/mate_1ph_piline  FF=60  conf=config 11  lenfeet=250  dmi=off  RR1=0.8  LL1=0.002  CC1=7e-9  lenkm=1
  scc_1ph_piline24 : simetranss/Lines/mate_1ph_piline  FF=60  conf=config 11  lenfeet=200  dmi=off  RR1=0.8  LL1=0.002  CC1=7e-9  lenkm=1
  scc_1ph_piline25 : simetranss/Lines/mate_1ph_piline  FF=60  conf=config 11  lenfeet=325  dmi=off  RR1=0.8  LL1=0.002  CC1=7e-9  lenkm=1
  scc_1ph_piline26 : simetranss/Lines/mate_1ph_piline  FF=60  conf=config 11  lenfeet=250  dmi=off  RR1=0.8  LL1=0.002  CC1=7e-9  lenkm=1
  scc_1ph_piline27 : simetranss/Lines/mate_1ph_piline  FF=60  conf=config 10  lenfeet=225  dmi=off  RR1=0.8  LL1=0.002  CC1=7e-9  lenkm=1
  scc_1ph_piline28 : simetranss/Lines/mate_1ph_piline  FF=60  conf=config 11  lenfeet=150  dmi=off  RR1=0.8  LL1=0.002  CC1=7e-9  lenkm=1
  scc_1ph_piline29 : simetranss/Lines/mate_1ph_piline  FF=60  conf=config 11  lenfeet=100  dmi=off  RR1=0.8  LL1=0.002  CC1=7e-9  lenkm=1
  scc_1ph_piline3 : simetranss/Lines/mate_1ph_piline  FF=60  conf=config 10  lenfeet=225  dmi=off  RR1=0.8  LL1=0.002  CC1=7e-9  lenkm=300*ft2km
  scc_1ph_piline30 : simetranss/Lines/mate_1ph_piline  FF=60  conf=config 11  lenfeet=375  dmi=off  RR1=0.8  LL1=0.002  CC1=7e-9  lenkm=1
  scc_1ph_piline31 : simetranss/Lines/mate_1ph_piline  FF=60  conf=config 11  lenfeet=350  dmi=off  RR1=0.8  LL1=0.002  CC1=7e-9  lenkm=1
  scc_1ph_piline32 : simetranss/Lines/mate_1ph_piline  FF=60  conf=config 10  lenfeet=175  dmi=off  RR1=0.8  LL1=0.002  CC1=7e-9  lenkm=1
  scc_1ph_piline33 : simetranss/Lines/mate_1ph_piline  FF=60  conf=config 9  lenfeet=225  dmi=off  RR1=0.8  LL1=0.002  CC1=7e-9  lenkm=1
  scc_1ph_piline34 : simetranss/Lines/mate_1ph_piline  FF=60  conf=config 9  lenfeet=425  dmi=off  RR1=0.8  LL1=0.002  CC1=7e-9  lenkm=1
  scc_1ph_piline35 : simetranss/Lines/mate_1ph_piline  FF=60  conf=config 9  lenfeet=250  dmi=off  RR1=0.8  LL1=0.002  CC1=7e-9  lenkm=1
  scc_1ph_piline36 : simetranss/Lines/mate_1ph_piline  FF=60  conf=config 9  lenfeet=250  dmi=off  RR1=0.8  LL1=0.002  CC1=7e-9  lenkm=1
  scc_1ph_piline4 : simetranss/Lines/mate_1ph_piline  FF=60  conf=config 9  lenfeet=175  dmi=off  RR1=0.8  LL1=0.002  CC1=7e-9  lenkm=300*ft2km
  scc_1ph_piline51 : simetranss/Lines/mate_1ph_piline  FF=60  conf=config 10  lenfeet=250  dmi=off  RR1=0.8  LL1=0.002  CC1=7e-9  lenkm=300*ft2km
  scc_1ph_piline52 : simetranss/Lines/mate_1ph_piline  FF=60  conf=config 10  lenfeet=250  dmi=off  RR1=0.8  LL1=0.002  CC1=7e-9  lenkm=300*ft2km
  scc_3ph_piline : simetranss/Lines/mate_3ph_piline  FF=60  conf=config 1  lenfeet=400  dmi=off  RR33=[1 0 0;0 1 0; 0 0 1]  LL33=[1 0 0;0 1 0; 0 0 1]  CC33=[1 0 0;0 1 0; 0 0 1]  lenkm=1
  scc_3ph_piline1 : simetranss/Lines/mate_3ph_piline  FF=60  conf=config 1  lenfeet=300  dmi=off  RR33=[1 0 0;0 1 0; 0 0 1]  LL33=[1 0 0;0 1 0; 0 0 1]  CC33=[1 0 0;0 1 0; 0 0 1]  lenkm=1
  scc_3ph_piline10 : simetranss/Lines/mate_3ph_piline  FF=60  conf=config 6  lenfeet=225  dmi=off  RR33=[1 0 0;0 1 0; 0 0 1]  LL33=[1 0 0;0 1 0; 0 0 1]  CC33=[1 0 0;0 1 0; 0 0 1]  lenkm=1
  scc_3ph_piline11 : simetranss/Lines/mate_3ph_piline  FF=60  conf=config 6  lenfeet=225  dmi=off  RR33=[1 0 0;0 1 0; 0 0 1]  LL33=[1 0 0;0 1 0; 0 0 1]  CC33=[1 0 0;0 1 0; 0 0 1]  lenkm=1
  scc_3ph_piline12 : simetranss/Lines/mate_3ph_piline  FF=60  conf=config 6  lenfeet=275  dmi=off  RR33=[1 0 0;0 1 0; 0 0 1]  LL33=[1 0 0;0 1 0; 0 0 1]  CC33=[1 0 0;0 1 0; 0 0 1]  lenkm=1
  scc_3ph_piline13 : simetranss/Lines/mate_3ph_piline  FF=60  conf=config 6  lenfeet=400  dmi=off  RR33=[1 0 0;0 1 0; 0 0 1]  LL33=[1 0 0;0 1 0; 0 0 1]  CC33=[1 0 0;0 1 0; 0 0 1]  lenkm=1
  scc_3ph_piline2 : simetranss/Lines/mate_3ph_piline  FF=60  conf=config 1  lenfeet=200  dmi=off  RR33=[1 0 0;0 1 0; 0 0 1]  LL33=[1 0 0;0 1 0; 0 0 1]  CC33=[1 0 0;0 1 0; 0 0 1]  lenkm=1
  scc_3ph_piline3 : simetranss/Lines/mate_3ph_piline  FF=60  conf=config 1  lenfeet=300  dmi=off  RR33=[1 0 0;0 1 0; 0 0 1]  LL33=[1 0 0;0 1 0; 0 0 1]  CC33=[1 0 0;0 1 0; 0 0 1]  lenkm=1
  scc_3ph_piline4 : simetranss/Lines/mate_3ph_piline  FF=60  conf=config 1  lenfeet=400  dmi=off  RR33=[1 0 0;0 1 0; 0 0 1]  LL33=[1 0 0;0 1 0; 0 0 1]  CC33=[1 0 0;0 1 0; 0 0 1]  lenkm=1
  scc_3ph_piline48 : simetranss/Lines/mate_3ph_piline  FF=60  conf=config 3  lenfeet=350  dmi=off  RR33=[1 0 0;0 1 0; 0 0 1]  LL33=[1 0 0;0 1 0; 0 0 1]  CC33=[1 0 0;0 1 0; 0 0 1]  lenkm=1
  scc_3ph_piline5 : simetranss/Lines/mate_3ph_piline  FF=60  conf=config 1  lenfeet=200  dmi=off  RR33=[1 0 0;0 1 0; 0 0 1]  LL33=[1 0 0;0 1 0; 0 0 1]  CC33=[1 0 0;0 1 0; 0 0 1]  lenkm=1
  scc_3ph_piline6 : simetranss/Lines/mate_3ph_piline  FF=60  conf=config 1  lenfeet=125  dmi=off  RR33=[1 0 0;0 1 0; 0 0 1]  LL33=[1 0 0;0 1 0; 0 0 1]  CC33=[1 0 0;0 1 0; 0 0 1]  lenkm=1
  scc_3ph_piline7 : simetranss/Lines/mate_3ph_piline  FF=60  conf=config 1  lenfeet=275  dmi=off  RR33=[1 0 0;0 1 0; 0 0 1]  LL33=[1 0 0;0 1 0; 0 0 1]  CC33=[1 0 0;0 1 0; 0 0 1]  lenkm=1
  scc_3ph_piline8 : simetranss/Lines/mate_3ph_piline  FF=60  conf=config 1  lenfeet=275  dmi=off  RR33=[1 0 0;0 1 0; 0 0 1]  LL33=[1 0 0;0 1 0; 0 0 1]  CC33=[1 0 0;0 1 0; 0 0 1]  lenkm=1
  scc_3ph_piline9 : simetranss/Lines/mate_3ph_piline  FF=60  conf=config 6  lenfeet=300  dmi=off  RR33=[1 0 0;0 1 0; 0 0 1]  LL33=[1 0 0;0 1 0; 0 0 1]  CC33=[1 0 0;0 1 0; 0 0 1]  lenkm=1
  sph : Subsystem
  sph1 : Subsystem
  sph2 : Subsystem
  sph24 : Subsystem
  sph25 : Subsystem
  sph26 : Subsystem
  sph27 : Subsystem
  sph28 : Subsystem
  sph29 : Subsystem
  sph3 : Subsystem
  sph30 : Subsystem
  sph4 : Subsystem
  sph42 : Subsystem
  sph43 : Subsystem
  sph44 : Subsystem
  sph5 : Subsystem
  sph51 : Subsystem
  sph6 : Subsystem
  sph7 : Subsystem
  sph8 : Subsystem
  P1 : PMIOPort  Side=Left
  P2 : PMIOPort  Port=2  Side=Right
  P3 : PMIOPort  Port=3  Side=Right
  connections:
  scc_1ph_piline24/LConn1 -- SPOT 4/LConn1
  scc_3ph_piline7/RConn1 -- 8/RConn1
  scc_3ph_piline2/RConn1 -- 2/RConn1 -- sph30/LConn1 -- sph26/LConn1
  scc_1ph_piline33/RConn1 -- scc_1ph_piline34/RConn1 -- SPOT 9/LConn1
  sph5/RConn1 -- scc_1ph_piline2/RConn1
  1/LConn1 -- scc_3ph_piline2/LConn1
  scc_3ph_piline4/RConn1 -- 4/RConn1
  scc_1ph_piline51/RConn1 -- SPOT 58/LConn1 -- scc_1ph_piline52/LConn1
  SPOT 86/LConn1 -- sph2/RConn1
  sph6/RConn1 -- scc_1ph_piline1/RConn1
  scc_1ph_piline26/RConn1 -- SPOT 6/LConn1
  sph29/RConn1 -- SPOT 7/LConn1
  scc_3ph_piline1/LConn1 -- sph24/LConn1 -- 5/LConn1 -- sph28/LConn1
  SPOT 88/LConn1 -- SimScape 1ph C load/LConn1 -- scc_1ph_piline4/LConn1
  7/LConn1 -- scc_3ph_piline48/RConn1 -- scc_3ph_piline7/LConn1
  scc_3ph_piline9/RConn1 -- 10/RConn1 -- sph6/LConn1
  scc_1ph_piline23/LConn1 -- 21/RConn1 -- scc_1ph_piline24/RConn1
  SPOT 56/LConn1 -- sph/RConn1
  4/LConn1 -- sph43/LConn1 -- scc_3ph_piline5/LConn1
  scc_1ph_piline35/LConn1 -- SPOT 11/LConn1
  scc_3ph_piline8/RConn1 -- 9/RConn1
  MATE 3ph/LConn1 -- P1/RConn1
  SPOT 95/LConn1 -- sph3/RConn1
  scc_1ph_piline31/RConn1 -- SPOT 2/LConn1
  scc_1ph_piline33/LConn1 -- sph30/RConn1
  scc_1ph_piline29/RConn1 -- scc_1ph_piline30/LConn1 -- 22/LConn1
  scc_3ph_piline6/RConn1 -- 7/RConn1 -- sph51/LConn1
  8/LConn1 -- scc_3ph_piline8/LConn1
  scc_3ph_piline10/RConn1 -- 11/RConn1 -- sph5/LConn1
  sph4/RConn1 -- scc_1ph_piline/RConn1
  scc_3ph_piline5/RConn1 -- 6/RConn1 -- sph44/LConn1
  scc_1ph_piline26/LConn1 -- SPOT 5/LConn1 -- scc_1ph_piline25/RConn1
  scc_3ph_piline10/LConn1 -- 10/LConn1
  scc_1ph_piline29/LConn1 -- SPOT 23/LConn1 -- scc_1ph_piline28/RConn1
  scc_1ph_piline28/LConn1 -- sph27/RConn1
  SPOT 87/LConn1 -- sph1/RConn1
  scc_3ph_piline11/RConn1 -- 12/RConn1 -- sph7/LConn1
  scc_3ph_piline1/RConn1 -- sph29/LConn1 -- 1/RConn1
  sph25/RConn1 -- SPOT 1./LConn1
  sph26/RConn1 -- scc_1ph_piline27/LConn1
  SPOT 12/LConn1 -- scc_1ph_piline27/RConn1
  sph8/RConn1 -- scc_1ph_piline4/RConn1
  sph24/RConn1 -- scc_1ph_piline23/RConn1
  scc_1ph_piline25/LConn1 -- 21/LConn1
  22/RConn1 -- scc_1ph_piline31/LConn1
  scc_3ph_piline13/RConn1 -- MATE 3ph2/RConn1 -- sph2/LConn1
  scc_1ph_piline32/RConn1 -- SPOT 2./LConn1
  Nonlinear Transformer/RConn2 -- Electrical Reference/LConn1
  Nonlinear Transformer/LConn2 -- Electrical Reference1/LConn1
  scc_1ph_piline/LConn1 -- SPOT 96/LConn1
  Electrical Reference2/LConn1 -- Solver Configuration/RConn1 -- Voltage Source (Three-Phase)1/LConn1
  scc_1ph_piline52/RConn1 -- SPOT 59/LConn1
  34/LConn1 -- sph42/LConn1
  5/RConn1 -- sph25/LConn1 -- scc_3ph_piline/RConn1
  scc_1ph_piline36/RConn1 -- SPOT 10/LConn1
  scc_1ph_piline51/LConn1 -- sph42/RConn1
  scc_1ph_piline32/LConn1 -- sph28/RConn1
  SPOT 53/LConn1 -- sph44/RConn1
  SPOT 52/LConn1 -- sph43/RConn1
  scc_1ph_piline30/RConn1 -- SPOT 16/LConn1
  scc_1ph_piline35/RConn1 -- scc_1ph_piline36/LConn1 -- 23/RConn1
  sph51/RConn1 -- MATE Breaker/LConn1
  scc_1ph_piline2/LConn1 -- SimScape 1ph C load1/LConn1 -- SPOT 92/LConn1
  scc_1ph_piline1/LConn1 -- SPOT 94/LConn1 -- MATE Breaker/RConn1
  11/LConn1 -- scc_3ph_piline11/LConn1
  2/LConn1 -- scc_3ph_piline3/LConn1
  scc_3ph_piline12/LConn1 -- 12/LConn1
  scc_3ph_piline3/RConn1 -- 3/RConn1
  6/LConn1 -- scc_3ph_piline6/LConn1
  sph7/RConn1 -- scc_1ph_piline3/RConn1
  scc_1ph_piline3/LConn1 -- SimScape 1ph C load2/LConn1 -- SPOT 90/LConn1
  scc_3ph_piline13/LConn1 -- sph1/LConn1 -- sph8/LConn1 -- scc_3ph_piline12/RConn1
  9/LConn1 -- sph/LConn1
  scc_3ph_piline9/LConn1 -- sph3/LConn1 -- sph4/LConn1
  r1/LConn1 -- MATE 3ph/RConn1 -- 3/LConn1 -- sph27/LConn1
  MATE 3ph1/LConn1 -- P2/RConn1
  MATE 3ph2/LConn1 -- P3/RConn1
  23/LConn1 -- Nonlinear Transformer/LConn1
  scc_1ph_piline34/LConn1 -- Nonlinear Transformer/RConn1
  MATE 3ph Breaker/RConn1 -- scc_3ph_piline4/LConn1
  MATE 3ph Breaker/LConn1 -- bus13VI/RConn1
  Two-Winding Transformer 115/4.16 kV (Three-Phase) D-Yg2/LConn1 -- Voltage Source (Three-Phase)1/RConn1
  RLC (Three-Phase)1/RConn1 -- MATE 3ph1/RConn1
  scc_3ph_piline48/LConn1 -- RLC (Three-Phase)1/LConn1 -- 34/RConn1
  r1/RConn1 -- bus13VI/LConn1
  Two-Winding Transformer 115/4.16 kV (Three-Phase) D-Yg2/RConn1 -- CV_xfo/RConn1
  CV_xfo/LConn1 -- scc_3ph_piline/LConn1

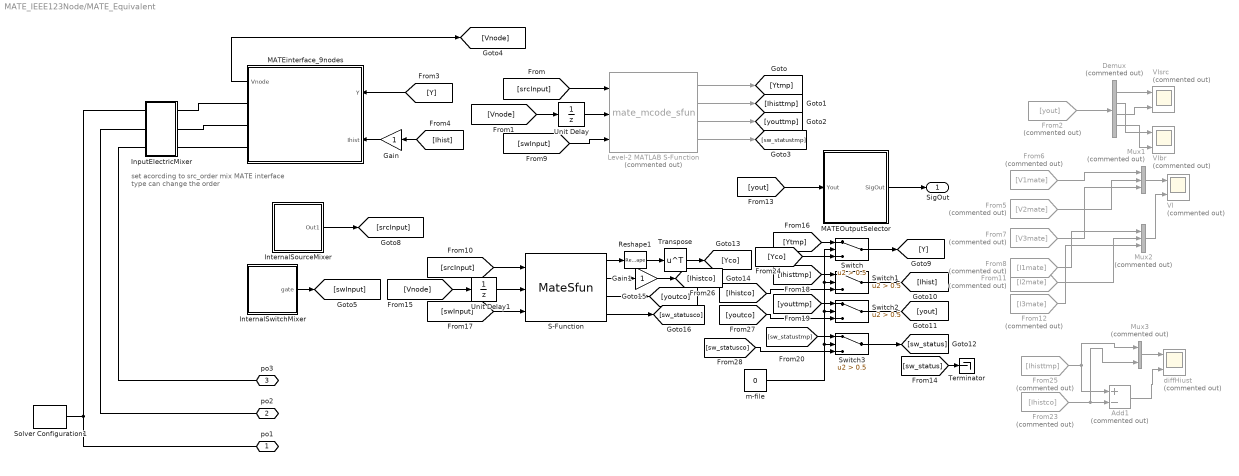
== system MATE_IEEE123Node/MATE_Equivalent ==
  note: set acorcding to src_order
      | mix MATE interface type can change the order
  Add1 : Sum  Commented=on  Inputs=+-
  Demux : Demux  Commented=on  Outputs=[4 3 3 3 3 9]
  From11 : From  Commented=on  GotoTag=I2mate  TagVisibility=global
  From12 : From  Commented=on  GotoTag=I3mate  TagVisibility=global
  From2 : From  Commented=on  GotoTag=yout
  From23 : From  Commented=on  GotoTag=Ihistco
  From25 : From  Commented=on  GotoTag=Ihisttmp
  From5 : From  Commented=on  GotoTag=V2mate  TagVisibility=global
  From6 : From  Commented=on  GotoTag=V1mate  TagVisibility=global
  From7 : From  Commented=on  GotoTag=V3mate  TagVisibility=global
  From8 : From  Commented=on  GotoTag=I1mate  TagVisibility=global
  Gain : Gain
  Gain1 : Gain
  InputElectricMixer : Subsystem
  InternalSourceMixer : Subsystem
  InternalSwitchMixer : Subsystem
  Level-2 MATLAB S-Function : M-S-Function  Commented=on  FunctionName=mate_mcode_sfun  Parameters=MATE
  MATEOutputSelector : Subsystem
  MATEinterface_9nodes : Subsystem
  Mux1 : Mux  Commented=on  Inputs=3
  Mux2 : Mux  Commented=on  Inputs=3
  Mux3 : Mux  Commented=on  Inputs=2
  Reshape1 : Reshape  OutputDimensionality=Customize  OutputDimensions=[MATE.NumberOfNodes,MATE.NumberOfNodes]
  S-Function : S-Function  FunctionName=MateSfun  Parameters="MATERT.sizes,MATERT.As  ,MATERT.Bs,MATERT.Cs,MATERT.Ds,MATERT.Rsw,MATERT.SwType,MATERT.DISC,MATERT.h,MATERT.U0,MATERT.X0,MATERT.SwitchVf"  SFunctionDeploymentMode=off  EnableBusSupport=off
  Solver Configuration1 : nesl_utility/Solver Configuration  PhysicalDomain=network_engine_domain  SubClassName=solver  LeftPortType=input  RightPortType=generic  Tones=[]  Harmonics=[]  SimulateNoise=off  Profile=off  UseLocalSampling=off  EnableSwitchedLinearOptims=on  FrequencyDomain=off  UseCCode=off  RelTol=0.001  AbsTol=0.001  MinStep=1e-09  ToWorkspace=off  RevertToSquareIcSolve=off  NumHomotopyIterations=100  PhasorMode=off  PhasorModeNumHarmonics=1  ConsistencySolver=NEWTON_XTOL_AFTER_FTOL  IndexReductionMethod=DerivativeReplacement  DoDC=off  ResidualTolerance=1e-09  ConsistencyTolSource=GLOBAL  ConsistencyAbsTol=0.001  ConsistencyRelTol=0.001  ConsistencyTolFactor=0.001  UseLocalSolver=on  LocalSolverChoice=NE_BACKWARD_EULER_ADVANCER  ResolveIndetEquations=off  FunctionEvalNumThread=1  LocalSolverSampleTime=Ts  DoFixedCost=on  MaxNonlinIter=1  MaxModeIter=2  ComputeImpulses=off  ImpulseIterations=2  LinearAlgebra=auto  LinearAlgebraNumThread=0  EquationFormulation=NE_TIME_EF  DelaysMemoryBudget=1024  AutomaticFiltering=off  FilteringTimeConstant=0.001  PartitionStorageMethod=AS_NEEDED  PartitionMemoryBudget=1024  PartitionMethod=ROBUST  MultibodyUseLocalSolver=off  MultibodyLocalSolverChoice=ODE1  MultibodyLocalSolverSampleTime=0.001
  Switch{,1..3} (4 alike) : Switch  Criteria=u2 > Threshold  Threshold=0.5  SaturateOnIntegerOverflow=off  InputSameDT=off
  Terminator : Terminator
  Transpose : Math  Operator=transpose
  Unit Delay : UnitDelay  SampleTime=Ts  HasFrameUpgradeWarning=on
  Unit Delay1 : UnitDelay  SampleTime=Ts  HasFrameUpgradeWarning=on
  VI : Scope  Commented=on  NumInputPorts=2
  VIbr : Scope  Commented=on  NumInputPorts=2
  VIsrc : Scope  Commented=on  NumInputPorts=2
  diffHiust : Scope  Commented=on  NumInputPorts=2
  m-file : Constant  Value=0
  po1 : PMIOPort  Side=Left
  po2 : PMIOPort  Port=2  Side=Right
  po3 : PMIOPort  Port=3  Side=Right
  SigOut : Outport
  wires:
  [Yco] -> Switch/3
  S-Function/1 -> Reshape1/1
  Switch1/1 -> [Ihist]
  Add1/1 -> diffHiust/2
  From25/1 -> Mux3/1, Add1/1
  From23/1 -> Mux3/2, Add1/2
  S-Function/4 -> [sw_statusco]
  Reshape1/1 -> Transpose/1
  [Ihistco] -> Switch1/3
  [youtco] -> Switch2/3
  InternalSwitchMixer/1(gate) -> [swInput]
  InternalSourceMixer/1(Out1) -> [srcInput]
  S-Function/3 -> [youtco]
  Level-2 MATLAB S-Function/3 -> [youttmp]
  Gain1/1 -> [Ihistco]
  [Ytmp] -> Switch/1
  [sw_statustmp] -> Switch3/1
  [Ihisttmp] -> Switch1/1
  Unit Delay/1 -> Level-2 MATLAB S-Function/2
  Switch2/1 -> [yout]
  Unit Delay1/1 -> S-Function/2
  [Vnode] -> Unit Delay1/1
  [sw_statusco] -> Switch3/3
  Transpose/1 -> [Yco]
  [Vnode] -> Unit Delay/1
  Switch3/1 -> [sw_status]
  [srcInput] -> S-Function/1
  Gain/1 -> MATEinterface_9nodes/2(Ihist)
  Level-2 MATLAB S-Function/1 -> [Ytmp]
  [Ihist] -> Gain/1
  Level-2 MATLAB S-Function/2 -> [Ihisttmp]
  Level-2 MATLAB S-Function/4 -> [sw_statustmp]
  Switch/1 -> [Y]
  Mux3/1 -> diffHiust/1
  MATEinterface_9nodes/1(Vnode) -> [Vnode]
  [youttmp] -> Switch2/1
  S-Function/2 -> Gain1/1
  [Y] -> MATEinterface_9nodes/1(Y)
  m-file/1 -> Switch3/2, Switch/2, Switch1/2, Switch2/2
  Mux1/1 -> VI/1
  From5/1 -> Mux1/2
  From6/1 -> Mux1/1
  From7/1 -> Mux1/3
  From8/1 -> Mux2/1
  From11/1 -> Mux2/2
  From12/1 -> Mux2/3
  Mux2/1 -> VI/2
  [srcInput] -> Level-2 MATLAB S-Function/1
  [swInput] -> S-Function/3
  [swInput] -> Level-2 MATLAB S-Function/3
  From2/1 -> Demux/1
  Demux/2 -> VIsrc/1
  Demux/4 -> VIsrc/2
  Demux/3 -> VIbr/1
  Demux/5 -> VIbr/2
  [yout] -> MATEOutputSelector/1(Yout)
  MATEOutputSelector/1(SigOut) -> SigOut/1
  [sw_status] -> Terminator/1
  connections:
  InputElectricMixer/LConn2 -- po2/RConn1
  InputElectricMixer/LConn1 -- po1/RConn1 -- Solver Configuration1/RConn1
  InputElectricMixer/LConn3 -- po3/RConn1
  InputElectricMixer/RConn1 -- MATEinterface_9nodes/RConn1
  InputElectricMixer/RConn2 -- MATEinterface_9nodes/RConn2
  InputElectricMixer/RConn3 -- MATEinterface_9nodes/RConn3
